simulink model "Block_Daigram_open_loop_turbulence"  (R2016a)
settings: Solver=ode45  StartTime=0.0  StopTime=50  RelTol=1e-3
settings Model: Creator=Muhammad Zubair  LastModifiedBy=Muhammad Zubair

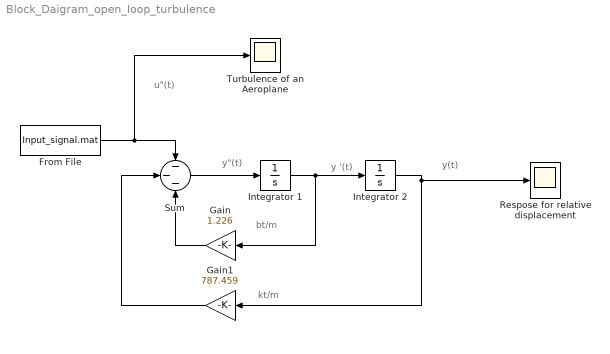
== system Block_Daigram_open_loop_turbulence ==
  note: u"(t)
  note: kt/m
  note: bt/m
  note: y(t)
  note: y '(t)
  note: y"(t)
  From File : FromFile  FileName=Input_signal.mat  SampleTime=0
  Gain : Gain  Gain=1.226
  Gain1 : Gain  Gain=787.459
  Integrator 1 : Integrator
  "Integrator 2 " : Integrator
  Respose for relative displacement : Scope
  Sum : Sum  Inputs=---
  Turbulence of an Aeroplane : Scope
  wires:
  Sum/1 -> Integrator 1/1
  Integrator 1/1 -> Gain/1, "Integrator 2 "/1
  Gain/1 -> Sum/3
  Gain1/1 -> Sum/2
  "Integrator 2 "/1 -> Respose for relative displacement/1, Gain1/1
  From File/1 -> Sum/1, Turbulence of an Aeroplane/1
